simulink model "E_Netzwerk"  (R2017b)
settings: Solver=ode45  StartTime=0.0  StopTime=10.0  RelTol=1e-3
values from neighbouring files (symbols this model uses):
  C1_ref = 1e-6    (= 1e-06)    [Esys_Parameter.m]
  C2 = 1e-6    (= 1e-06)    [Esys_Parameter.m]
  K = 3    [Esys_Parameter.m]
  kC1 = 800e-9    (= 8e-07)    [Esys_Parameter.m]
  R_1 = 625    [Esys_Parameter.m]
  R_2 = 3500    [Esys_Parameter.m]
  te = .05    (= 0.05)    [Esys_Parameter.m]
  ts = .1    (= 0.1)    [Esys_Parameter.m]
  UC1_ref = -10    [Esys_Parameter.m]
  Ue = 7    [Esys_Parameter.m]
  UeR = 5    [Esys_Parameter.m]
  Us = 4    [Esys_Parameter.m]
  Usinus = 1    [Esys_Parameter.m]
  UsR = 5    [Esys_Parameter.m]
  we = 1000    [Esys_Parameter.m]
undefined symbols (not defined in the file or in its folder): k, UC1R, UC2R
libraries: cstblocks x4, simulink x1
settings Model: Creator=sj  LastModifiedBy=Alexander Aschauer
settings DataIOCC: LimitDataPoints=on  SaveFormat=Array
settings OptimizationCC: BlockReduction=off  BooleanDataType=off  LifeSpan=inf
settings DebuggingCC: SaveWithParameterizedLinksMsg=none  UnderspecifiedInitializationDetection=Classic  MergeDetectMultiDrivingBlocksExec=none  SignalResolutionControl=TryResolveAllWithWarning  StrictBusMsg=Warning  SFUnexpectedBacktrackingDiag=warning  SFNoUnconditionalDefaultTransitionDiag=warning  SFExecutionAtInitializationDiag=none
settings HardwareCC: ProdBitPerPointer=32  ProdBitPerSizeT=32  ProdBitPerPtrDiffT=32  ProdLargestAtomicFloat=None  ProdIntDivRoundTo=Undefined  ProdEndianess=Unspecified  ProdWordSize=32  ProdHWDeviceType=32-bit Generic  TargetUnknown=on
settings ModelReferenceCC: PropagateSignalLabelsOutOfModel=off
settings CodeAppCC: StateflowObjectComments=on
settings GRTTargetCC: TargetLangStandard=C89/C90 (ANSI)  GeneratePreprocessorConditionals=Disable all
settings ConfigComp: CovMetricSettings=dw  CovHtmlReporting=on  CovSaveCumulativeToWorkspaceVar=on  CovSaveSingleToWorkspaceVar=on  CovExternalEMLEnable=off  CovSFcnEnable=off

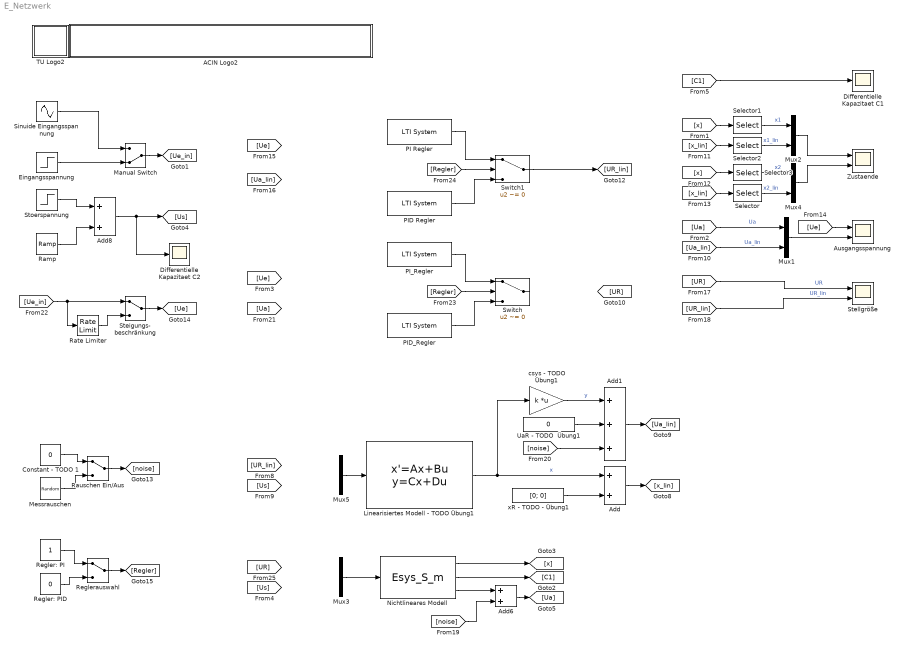
== system E_Netzwerk ==
  ACIN Logo2 : Subsystem
      mask init:
      | s = get_param(gcb,'UserData');
      mask Display:
      | image(s.logo,[0 0 439 45]);
      | %axis image
  Add : Sum
  Add1 : Sum  Inputs=+++
  Add6 : Sum
  Add8 : Sum
  Ausgangsspannung : Scope  NumInputPorts=2
  Constant - TODO 1 : Constant  Value=0
  Differentielle Kapazitaet C1 : Scope
  Differentielle Kapazitaet C2 : Scope
  Eingangsspannung : Step  Time=te  Before=UeR  After=Ue  SampleTime=0
  Linearisiertes Modell - TODO Übung1 : StateSpace  A=zeros(2)  B=zeros(2)  C=zeros(2)  D=zeros(2)  InitialCondition=[0;0]
  Manual Switch : ManualSwitch  CurrentSetting=0
  Messrauschen : UniformRandomNumber  Minimum=-5e-2  Maximum=5e-2  SampleTime=1e-3
  Mux{1..5} (5 alike) : Mux  Inputs=2
  Nichtlineares Modell : M-S-Function  FunctionName=Esys_S_m  Parameters=UC1R,UC2R,R_1,R_2,K,C1_ref,UC1_ref,kC1,C2
  PI Regler : cstblocks/LTI System  sys=tf(1,[1 1])  IC=[]
  PID Regler : cstblocks/LTI System  sys=tf(1,[1 1])  IC=[]
  PID_Regler : cstblocks/LTI System  sys=tf(1,[1 1])  IC=[]
  PI_Regler : cstblocks/LTI System  sys=tf(1,[1 1])  IC=[]
  Ramp : simulink/Sources/Ramp  slope=1  start=0  X0=0
  Rate Limiter : RateLimiter  RisingSlewLimit=100  FallingSlewLimit=-100  SampleTimeMode=inherited
  Rauschen Ein/Aus : ManualSwitch
  Regler: PI : Constant
  Regler: PID : Constant  Value=0
  Reglerauswahl : ManualSwitch
  Selector : Selector  InputPortWidth=2  IndexOptions=Index vector (dialog)  Indices=2  OutputSizes=1
  Selector1 : Selector  InputPortWidth=2  IndexOptions=Index vector (dialog)  Indices=1  OutputSizes=1
  Selector2 : Selector  InputPortWidth=2  IndexOptions=Index vector (dialog)  Indices=1  OutputSizes=1
  Selector3 : Selector  InputPortWidth=2  IndexOptions=Index vector (dialog)  Indices=2  OutputSizes=1
  Sinuide Eingangsspannung : Sin  Amplitude=Usinus  Bias=UeR  Frequency=we  SampleTime=0
  Steigungs- beschränkung : ManualSwitch
  Stellgröße : Scope  NumInputPorts=2
  Stoerspannung : Step  Time=ts  Before=UsR  After=Us  SampleTime=0
  Switch : Switch  Criteria=u2 ~= 0
  Switch1 : Switch  Criteria=u2 ~= 0
  TU Logo2 : Subsystem
      mask init:
      | s = get_param(gcb,'UserData');
      mask Display: image(s.logo,[0 0 45 45]);
  UaR - TODO  Übung1 : Constant  Value=0
  Zustaende : Scope  NumInputPorts=2
  csys - TODO Übung1 : Gain  Gain=k  Multiplication=Matrix(K*u)
  xR - TODO - Übung1 : Constant  Value=[0; 0]
  wires:
  Nichtlineares Modell/1 -> [x]
  Nichtlineares Modell/2 -> [C1]
  Eingangsspannung/1 -> Manual Switch/2
  Sinuide Eingangsspannung/1 -> Manual Switch/1
  Manual Switch/1 -> [Ue_in]
  [C1] -> Differentielle Kapazitaet C1/1
  Linearisiertes Modell - TODO Übung1/1 -> csys - TODO Übung1/1, Add/1  "x"
  Mux5/1 -> Linearisiertes Modell - TODO Übung1/1
  Add/1 -> [x_lin]
  xR - TODO - Übung1/1 -> Add/2
  csys - TODO Übung1/1 -> Add1/1  "y"
  Add1/1 -> [Ua_lin]
  [Ua] -> Mux1/1  "Ua"
  [Ua_lin] -> Mux1/2  "Ua_lin"
  Selector1/1 -> Mux2/1  "x1"
  Selector2/1 -> Mux2/2  "x1_lin"
  [x] -> Selector1/1
  [x_lin] -> Selector2/1
  Selector3/1 -> Mux4/1  "x2"
  Selector/1 -> Mux4/2  "x2_lin"
  [x] -> Selector3/1
  [x_lin] -> Selector/1
  Mux2/1 -> Zustaende/1
  Mux4/1 -> Zustaende/2
  [Ue] -> Ausgangsspannung/1
  Mux1/1 -> Ausgangsspannung/2
  [UR] -> Stellgröße/1  "UR"
  [UR_lin] -> Stellgröße/2  "UR_lin"
  ? -> PI_Regler/1, PID_Regler/1
  Mux3/1 -> Nichtlineares Modell/1
  Messrauschen/1 -> Rauschen Ein/Aus/2
  Constant - TODO 1/1 -> Rauschen Ein/Aus/1
  Rauschen Ein/Aus/1 -> [noise]
  Add6/1 -> [Ua]
  Nichtlineares Modell/3 -> Add6/1
  [noise] -> Add6/2
  [noise] -> Add1/3
  Steigungs- beschränkung/1 -> [Ue]
  [Ue_in] -> Rate Limiter/1, Steigungs- beschränkung/1
  Rate Limiter/1 -> Steigungs- beschränkung/2
  PI_Regler/1 -> Switch/1
  [Regler] -> Switch/2
  Regler: PID/1 -> Reglerauswahl/2
  Regler: PI/1 -> Reglerauswahl/1
  Reglerauswahl/1 -> [Regler]
  PID_Regler/1 -> Switch/3
  PI Regler/1 -> Switch1/1
  [Regler] -> Switch1/2
  PID Regler/1 -> Switch1/3
  Switch1/1 -> [UR_lin]
  Stoerspannung/1 -> Add8/1
  Ramp/1 -> Add8/2
  Add8/1 -> Differentielle Kapazitaet C2/1, [Us]
  ? -> PI Regler/1, PID Regler/1
  UaR - TODO  Übung1/1 -> Add1/2

== system E_Netzwerk/ACIN Logo2 ==

== system E_Netzwerk/TU Logo2 ==
